simulink model "SimulinkModel"  (R2026a)
settings: Solver=ode23s  StopTime=5
values from neighbouring files (symbols this model uses):
  Kd = 2    [BaseSkript.m]
  Ki = 1.5    [BaseSkript.m]
  Kp = 40    [BaseSkript.m]
  Nd = 100    [BaseSkript.m]    (also in Master_Combination_Run.m; Master_Combination_Run_Prisme.m)
  s = 10*tau^3 - 15*tau^4 + 6*tau^5    [Math_Model.m]    (also in calculate_delta_torque.m = u^3 * (10 - 15*u + 6*u^2))
  X = P(1)*cos(phi_ang) + P(2)*sin(phi_ang)    [Math_Model.m]    (also in calculate_delta_torque.m = P(1)*cos(phi) + P(2)*sin(phi))
  Y = -P(1)*sin(phi_ang) + P(2)*cos(phi_ang)    [Math_Model.m]    (also in calculate_delta_torque.m = -P(1)*sin(phi) + P(2)*cos(phi))
  Z = P(3)    [Math_Model.m]    (also in calculate_delta_torque.m)
undefined symbols (not defined in the file or in its folder): params
libraries: sm_lib x17, nesl_utility x13, slpidlib x3
settings Model: Creator=louis  LastModifiedBy=louis

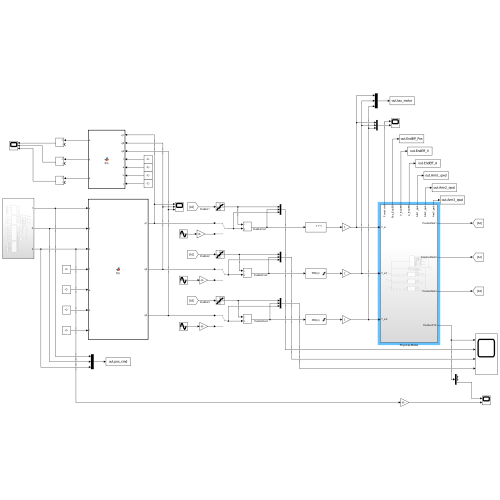
[thumbnail: Simulink's stored preview of the top-level diagram]
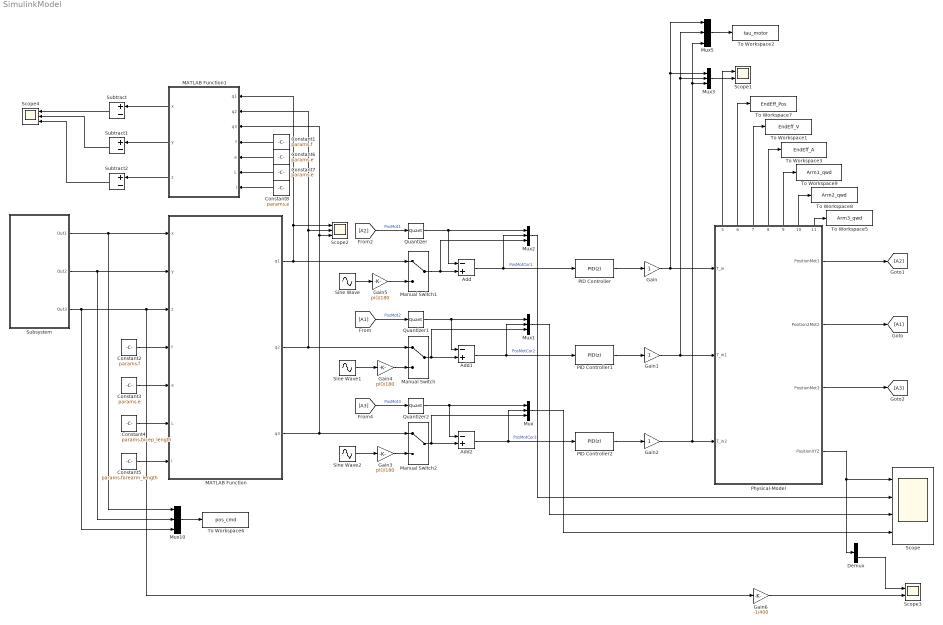
== system SimulinkModel ==
  Add : Sum  Inputs=-+
  Add1 : Sum  Inputs=-+
  Add2 : Sum  Inputs=-+
  Constant1 : Constant  Value=params.f
  Constant2 : Constant  Value=params.f
  Constant{3,6..8} (4 alike) : Constant  Value=params.e
  Constant4 : Constant  Value=params.bicep_length
  Constant5 : Constant  Value=params.forearm_length
  Demux : Demux  Outputs=3
  Gain : Gain
  Gain1 : Gain
  Gain2 : Gain
  Gain3 : Gain  Gain=pi()/180
  Gain4 : Gain  Gain=pi()/180
  Gain5 : Gain  Gain=pi()/180
  Gain6 : Gain  Gain=-1/400
  MATLAB Function : MATLAB Function  TreatAsAtomicUnit=on
  MATLAB Function1 : MATLAB Function  TreatAsAtomicUnit=on
  Manual Switch : ManualSwitch
  Manual Switch1 : ManualSwitch
  Manual Switch2 : ManualSwitch
  Mux{,1..3,5,10} (6 alike) : Mux  Inputs=3
  PID Controller : slpidlib/PID Controller  Controller=PID  Form=Parallel  TimeDomain=Discrete-time  UseExternalTs=off  SampleTime=0.001  IntegratorMethod=Forward Euler  FilterMethod=Forward Euler  ControllerParametersSource=internal  P=Kp  I=Ki  UseKiTs=off  D=Kd  UseExternalDerivativeSource=off  N=Nd  UseFilter=on  TunerSelectOption=Transfer Function Based (PID Tuner App)  InitialConditionSource=internal  InitialConditionForIntegrator=0  InitialConditionForFilter=0  DifferentiatorICPrevScaledInput=0  ExternalReset=none  TrackingMode=off  Kt=1  LimitOutput=on  SatLimitsSource=internal  UpperSaturationLimit=params.saturation_tau  LowerSaturationLimit=-params.saturation_tau  LinearizeAsGain=on  AntiWindupMode=none  Kb=1  LimitIntegrator=off  UpperIntegratorSaturationLimit=inf  LowerIntegratorSaturationLimit=-inf  POutMin=[]  POutMax=[]  IOutMin=[]  IOutMax=[]  DOutMin=[]  DOutMax=[]  NOutMin=[]  NOutMax=[]  SumOutMin=[]  SumOutMax=[]  SaturationOutMin=[]  SaturationOutMax=[]  PParamMin=[]  PParamMax=[]  IParamMin=[]  IParamMax=[]  DParamMin=[]  DParamMax=[]  NParamMin=[]  NParamMax=[]  KbParamMin=[]  KbParamMax=[]  KtParamMin=[]  KtParamMax=[]  KbOutMin=[]  KbOutMax=[]  KtOutMin=[]  KtOutMax=[]  IntegratorOutMin=[]  IntegratorOutMax=[]  FilterOutMin=[]  FilterOutMax=[]  SumI1OutMin=[]  SumI1OutMax=[]  SumI2OutMin=[]  SumI2OutMax=[]  SumI3OutMin=[]  SumI3OutMax=[]  SumI4OutMin=[]  SumI4OutMax=[]  SumDOutMin=[]  SumDOutMax=[]  DifferentiatorOutMin=[]  DifferentiatorOutMax=[]  FilterDiffOutCoefMin=[]  FilterDiffOutCoefMax=[]  ReciprocalOutMin=[]  ReciprocalOutMax=[]  SumDenOutMin=[]  SumDenOutMax=[]  SumNumOutMin=[]  SumNumOutMax=[]  DivideOutMin=[]  DivideOutMax=[]  UdiffTsProdOutMin=[]  UdiffTsProdOutMax=[]  NTsProdOutMin=[]  NTsProdOutMax=[]  UintegralTsProdOutMin=[]  UintegralTsProdOutMax=[]  UngainTsProdOutMin=[]  UngainTsProdOutMax=[]  ClampingZeroOutDataTypeStr=Inherit: Inherit via back propagation  ClampingZeroOutMin=[]  ClampingZeroOutMax=[]  FilterDenConstantOutDataTypeStr=Inherit: Inherit via back propagation  FilterDenConstantOutMin=[]  FilterDenConstantOutMax=[]  PCopyOutDataTypeStr=Inherit: Inherit via back propagation  PCopyOutMin=[]  PCopyOutMax=[]  NCopyOutDataTypeStr=Inherit: Inherit via back propagation  NCopyOutMin=[]  NCopyOutMax=[]  IntegratorContinuousStateAttributes=''  IntegratorStateMustResolveToSignalObject=off  IntegratorRTWStateStorageClass=Auto  FilterContinuousStateAttributes=''  FilterStateMustResolveToSignalObject=off  FilterRTWStateStorageClass=Auto  ParallelPVariant=InternalParameters  IdealPVariant=Disabled  IVariant=InternalParameters  DVariant=InternalParameters  IntegratorVariant=Discrete  SatVariant=Enabled  AWVariant=Passthrough  PCopyVariant=Disabled  TRVariant=Disabled  FdbkBlocksVariant=Forward  IdealPFdbkVariant=Disabled  SatFdbkVariant=Disabled  DerivativeFilterVariant=ForwardEulerFilter  NVariant=InternalParameters  NCopyVariant=Disabled  FilterICVariant=InternalICsFilter  IntegratorICVariant=InternalICs  ExternalResetVariant=Disabled  TRSumVariant=Passthrough  SumFdbkVariant=Disabled  SumVariant=Sum_PID  TsampFilterVariant=InternalTs  TsampNgainVariant=Passthrough  TsampIntegralVariant=Disabled_SignalSpec  ExternalSaturationOutDataTypeStr=Inherit: Same as second input  DerivativeSourceVariant=ErrorSignal  PreIntVariant=InternalPreInt
  PID Controller1 : slpidlib/PID Controller  Controller=PID  Form=Parallel  TimeDomain=Discrete-time  UseExternalTs=off  SampleTime=0.001  IntegratorMethod=Forward Euler  FilterMethod=Forward Euler  ControllerParametersSource=internal  P=Kp  I=Ki  UseKiTs=off  D=Kd  UseExternalDerivativeSource=off  N=Nd  UseFilter=on  TunerSelectOption=Transfer Function Based (PID Tuner App)  InitialConditionSource=internal  InitialConditionForIntegrator=0  InitialConditionForFilter=0  DifferentiatorICPrevScaledInput=0  ExternalReset=none  TrackingMode=off  Kt=1  LimitOutput=on  SatLimitsSource=internal  UpperSaturationLimit=params.saturation_tau  LowerSaturationLimit=-params.saturation_tau  LinearizeAsGain=on  AntiWindupMode=none  Kb=1  LimitIntegrator=off  UpperIntegratorSaturationLimit=inf  LowerIntegratorSaturationLimit=-inf  POutMin=[]  POutMax=[]  IOutMin=[]  IOutMax=[]  DOutMin=[]  DOutMax=[]  NOutMin=[]  NOutMax=[]  SumOutMin=[]  SumOutMax=[]  SaturationOutMin=[]  SaturationOutMax=[]  PParamMin=[]  PParamMax=[]  IParamMin=[]  IParamMax=[]  DParamMin=[]  DParamMax=[]  NParamMin=[]  NParamMax=[]  KbParamMin=[]  KbParamMax=[]  KtParamMin=[]  KtParamMax=[]  KbOutMin=[]  KbOutMax=[]  KtOutMin=[]  KtOutMax=[]  IntegratorOutMin=[]  IntegratorOutMax=[]  FilterOutMin=[]  FilterOutMax=[]  SumI1OutMin=[]  SumI1OutMax=[]  SumI2OutMin=[]  SumI2OutMax=[]  SumI3OutMin=[]  SumI3OutMax=[]  SumI4OutMin=[]  SumI4OutMax=[]  SumDOutMin=[]  SumDOutMax=[]  DifferentiatorOutMin=[]  DifferentiatorOutMax=[]  FilterDiffOutCoefMin=[]  FilterDiffOutCoefMax=[]  ReciprocalOutMin=[]  ReciprocalOutMax=[]  SumDenOutMin=[]  SumDenOutMax=[]  SumNumOutMin=[]  SumNumOutMax=[]  DivideOutMin=[]  DivideOutMax=[]  UdiffTsProdOutMin=[]  UdiffTsProdOutMax=[]  NTsProdOutMin=[]  NTsProdOutMax=[]  UintegralTsProdOutMin=[]  UintegralTsProdOutMax=[]  UngainTsProdOutMin=[]  UngainTsProdOutMax=[]  ClampingZeroOutDataTypeStr=Inherit: Inherit via back propagation  ClampingZeroOutMin=[]  ClampingZeroOutMax=[]  FilterDenConstantOutDataTypeStr=Inherit: Inherit via back propagation  FilterDenConstantOutMin=[]  FilterDenConstantOutMax=[]  PCopyOutDataTypeStr=Inherit: Inherit via back propagation  PCopyOutMin=[]  PCopyOutMax=[]  NCopyOutDataTypeStr=Inherit: Inherit via back propagation  NCopyOutMin=[]  NCopyOutMax=[]  IntegratorContinuousStateAttributes=''  IntegratorStateMustResolveToSignalObject=off  IntegratorRTWStateStorageClass=Auto  FilterContinuousStateAttributes=''  FilterStateMustResolveToSignalObject=off  FilterRTWStateStorageClass=Auto  ParallelPVariant=InternalParameters  IdealPVariant=Disabled  IVariant=InternalParameters  DVariant=InternalParameters  IntegratorVariant=Discrete  SatVariant=Enabled  AWVariant=Passthrough  PCopyVariant=Disabled  TRVariant=Disabled  FdbkBlocksVariant=Forward  IdealPFdbkVariant=Disabled  SatFdbkVariant=Disabled  DerivativeFilterVariant=ForwardEulerFilter  NVariant=InternalParameters  NCopyVariant=Disabled  FilterICVariant=InternalICsFilter  IntegratorICVariant=InternalICs  ExternalResetVariant=Disabled  TRSumVariant=Passthrough  SumFdbkVariant=Disabled  SumVariant=Sum_PID  TsampFilterVariant=InternalTs  TsampNgainVariant=Passthrough  TsampIntegralVariant=Disabled_SignalSpec  ExternalSaturationOutDataTypeStr=Inherit: Same as second input  DerivativeSourceVariant=ErrorSignal  PreIntVariant=InternalPreInt
  PID Controller2 : slpidlib/PID Controller  Controller=PID  Form=Parallel  TimeDomain=Discrete-time  UseExternalTs=off  SampleTime=0.001  IntegratorMethod=Forward Euler  FilterMethod=Forward Euler  ControllerParametersSource=internal  P=Kp  I=Ki  UseKiTs=off  D=Kd  UseExternalDerivativeSource=off  N=Nd  UseFilter=on  TunerSelectOption=Transfer Function Based (PID Tuner App)  InitialConditionSource=internal  InitialConditionForIntegrator=0.2  InitialConditionForFilter=0.2  DifferentiatorICPrevScaledInput=0  ExternalReset=none  TrackingMode=off  Kt=1  LimitOutput=on  SatLimitsSource=internal  UpperSaturationLimit=params.saturation_tau  LowerSaturationLimit=-params.saturation_tau  LinearizeAsGain=on  AntiWindupMode=none  Kb=1  LimitIntegrator=off  UpperIntegratorSaturationLimit=inf  LowerIntegratorSaturationLimit=-inf  POutMin=[]  POutMax=[]  IOutMin=[]  IOutMax=[]  DOutMin=[]  DOutMax=[]  NOutMin=[]  NOutMax=[]  SumOutMin=[]  SumOutMax=[]  SaturationOutMin=[]  SaturationOutMax=[]  PParamMin=[]  PParamMax=[]  IParamMin=[]  IParamMax=[]  DParamMin=[]  DParamMax=[]  NParamMin=[]  NParamMax=[]  KbParamMin=[]  KbParamMax=[]  KtParamMin=[]  KtParamMax=[]  KbOutMin=[]  KbOutMax=[]  KtOutMin=[]  KtOutMax=[]  IntegratorOutMin=[]  IntegratorOutMax=[]  FilterOutMin=[]  FilterOutMax=[]  SumI1OutMin=[]  SumI1OutMax=[]  SumI2OutMin=[]  SumI2OutMax=[]  SumI3OutMin=[]  SumI3OutMax=[]  SumI4OutMin=[]  SumI4OutMax=[]  SumDOutMin=[]  SumDOutMax=[]  DifferentiatorOutMin=[]  DifferentiatorOutMax=[]  FilterDiffOutCoefMin=[]  FilterDiffOutCoefMax=[]  ReciprocalOutMin=[]  ReciprocalOutMax=[]  SumDenOutMin=[]  SumDenOutMax=[]  SumNumOutMin=[]  SumNumOutMax=[]  DivideOutMin=[]  DivideOutMax=[]  UdiffTsProdOutMin=[]  UdiffTsProdOutMax=[]  NTsProdOutMin=[]  NTsProdOutMax=[]  UintegralTsProdOutMin=[]  UintegralTsProdOutMax=[]  UngainTsProdOutMin=[]  UngainTsProdOutMax=[]  ClampingZeroOutDataTypeStr=Inherit: Inherit via back propagation  ClampingZeroOutMin=[]  ClampingZeroOutMax=[]  FilterDenConstantOutDataTypeStr=Inherit: Inherit via back propagation  FilterDenConstantOutMin=[]  FilterDenConstantOutMax=[]  PCopyOutDataTypeStr=Inherit: Inherit via back propagation  PCopyOutMin=[]  PCopyOutMax=[]  NCopyOutDataTypeStr=Inherit: Inherit via back propagation  NCopyOutMin=[]  NCopyOutMax=[]  IntegratorContinuousStateAttributes=''  IntegratorStateMustResolveToSignalObject=off  IntegratorRTWStateStorageClass=Auto  FilterContinuousStateAttributes=''  FilterStateMustResolveToSignalObject=off  FilterRTWStateStorageClass=Auto  ParallelPVariant=InternalParameters  IdealPVariant=Disabled  IVariant=InternalParameters  DVariant=InternalParameters  IntegratorVariant=Discrete  SatVariant=Enabled  AWVariant=Passthrough  PCopyVariant=Disabled  TRVariant=Disabled  FdbkBlocksVariant=Forward  IdealPFdbkVariant=Disabled  SatFdbkVariant=Disabled  DerivativeFilterVariant=ForwardEulerFilter  NVariant=InternalParameters  NCopyVariant=Disabled  FilterICVariant=InternalICsFilter  IntegratorICVariant=InternalICs  ExternalResetVariant=Disabled  TRSumVariant=Passthrough  SumFdbkVariant=Disabled  SumVariant=Sum_PID  TsampFilterVariant=InternalTs  TsampNgainVariant=Passthrough  TsampIntegralVariant=Disabled_SignalSpec  ExternalSaturationOutDataTypeStr=Inherit: Same as second input  DerivativeSourceVariant=ErrorSignal  PreIntVariant=InternalPreInt
  Physical-Model : Subsystem
      settings: PortSchema="{\"entries\":[{\"content\":{\"sides\":[{\"content\":{\"connectorIds\":[\"In1\",\"In2\",\"In3\"]},\"type\":\"ConnectorPlacement.EquallySpacedRectSide\",\"uuid\":\"472b42dc-ef62-4194-8627-c0d485c40d23\"},{\"content\":{\"connectorIds\":[\"Out1\",\"Out2\",\"Out3\",\"Out4\"],\"side\":\"RIGHT\"},\"type\":\"ConnectorPlacement.EquallySpacedRectSide\",\"uuid\":\"1afa02f3-9060-449b-bf9c-19485df79b48\"},{\"content\":{\"connectorIds\":[\"Out5\",\"Out6\",\"Out7\",\"Out8\",\"Out9\",\"Out10\",\"Out11\"],\"side\":\"TOP\"},\"type\":\"ConnectorPlacement.EquallySpacedRectSide\",\"uuid\":\"4b06c459-0470-40e7-9b6b-03b6062bc28f\"}]},\"type\":\"ConnectorPlacement.EquallySpacedConnector\",\"uuid\":\"0d09a3c9-0e0a-4c94-88b6-5aaedb495534\"}],\"packageUris\":[\"http://schema.mathworks.com/mf0/Connector/R2020b\"],\"version\":\"1.0\"}"
  Quantizer : Quantizer  QuantizationInterval=(2*pi())/params.pulses_per_rev
  Quantizer1 : Quantizer  QuantizationInterval=(2*pi())/params.pulses_per_rev
  Quantizer2 : Quantizer  QuantizationInterval=(2*pi())/params.pulses_per_rev
  Scope : Scope  NumInputPorts=4
      settings: ActiveDisplayYMinimum=-0.346817893581086  ActiveDisplayYMaximum=0.17909621572480147
  Scope1 : Scope  NumInputPorts=2
      settings: ActiveDisplayYMinimum=-518.62097461648136  ActiveDisplayYMaximum=668.9682157183538
  Scope2 : Scope  NumInputPorts=3
      settings: ActiveDisplayYMinimum=0.80317985150487559  ActiveDisplayYMaximum=1.6546987147027221  DataLoggingVariableName=ScopeData2
  Scope3 : Scope  NumInputPorts=2
      settings: ActiveDisplayYMinimum=-0.36067756279258084  ActiveDisplayYMaximum=-0.28326753588358305  DataLoggingVariableName=ScopeData3
  Scope4 : Scope  NumInputPorts=3
      settings: ActiveDisplayYMinimum=-48.031147138395717  ActiveDisplayYMaximum=34.968785901954071  DataLoggingVariableName=ScopeData4
  Sine Wave : Sin  Amplitude=30  Bias=70  Frequency=2*pi()*2  Phase=(3/3) *( 2*pi())  SampleTime=0
  Sine Wave1 : Sin  Amplitude=30  Bias=70  Frequency=2*pi()*2  Phase=(1/3) *(2* pi())  SampleTime=0
  Sine Wave2 : Sin  Amplitude=30  Bias=70  Frequency=2*pi()*2  Phase=(2/3) *( 2*pi())  SampleTime=0
  Subsystem : Subsystem
  Subtract : Sum  Inputs=+-
  Subtract1 : Sum  Inputs=+-
  Subtract2 : Sum  Inputs=+-
  To Workspace1 : ToWorkspace  VariableName=EndEff_V  SaveFormat=Timeseries  SampleTime=-1
  To Workspace2 : ToWorkspace  VariableName=tau_motor  SaveFormat=Timeseries  SampleTime=-1
  To Workspace3 : ToWorkspace  VariableName=EndEff_A  SaveFormat=Timeseries  SampleTime=-1
  To Workspace5 : ToWorkspace  VariableName=Arm3_qwd  SaveFormat=Timeseries  SampleTime=-1
  To Workspace6 : ToWorkspace  VariableName=pos_cmd  SaveFormat=Timeseries  SampleTime=-1
  To Workspace7 : ToWorkspace  VariableName=EndEff_Pos  SaveFormat=Timeseries  SampleTime=-1
  To Workspace8 : ToWorkspace  VariableName=Arm2_qwd  SaveFormat=Timeseries  SampleTime=-1
  To Workspace9 : ToWorkspace  VariableName=Arm1_qwd  SaveFormat=Timeseries  SampleTime=-1
  wires:
  Add/1 -> PID Controller/1, Mux2/2  "PosMotCor1"
  Add2/1 -> PID Controller2/1, Mux/2  "PosMotCor3"
  Add1/1 -> PID Controller1/1, Mux1/2  "PosMotCor2"
  [A1] -> Quantizer1/1  "PosMot2"
  [A2] -> Quantizer/1  "PosMot1"
  [A3] -> Quantizer2/1  "PosMot3"
  Mux2/1 -> Scope/2
  Mux1/1 -> Scope/3
  Mux/1 -> Scope/4
  Constant3/1 -> MATLAB Function/5(e)
  Constant2/1 -> MATLAB Function/4(f)
  Constant4/1 -> MATLAB Function/6(L)
  Constant5/1 -> MATLAB Function/7(l)
  Gain/1 -> Physical-Model/1(T_in), Mux3/1, Mux5/1
  Gain1/1 -> Physical-Model/2(T_in1), Mux3/2, Mux5/2
  Gain2/1 -> Physical-Model/3(T_in2), Mux5/3, Mux3/3
  MATLAB Function/1(q1) -> MATLAB Function1/1(q1), Scope2/1, Manual Switch1/1
  MATLAB Function/3(q3) -> Manual Switch2/1, MATLAB Function1/3(q3), Scope2/3
  MATLAB Function/2(q2) -> Manual Switch/1, MATLAB Function1/2(q2), Scope2/2
  PID Controller/1 -> Gain/1
  PID Controller1/1 -> Gain1/1
  Sine Wave/1 -> Gain5/1
  Sine Wave1/1 -> Gain4/1
  Sine Wave2/1 -> Gain3/1
  PID Controller2/1 -> Gain2/1
  Gain4/1 -> Manual Switch/2
  Manual Switch1/1 -> Mux2/3, Add/2
  Gain5/1 -> Manual Switch1/2
  Manual Switch2/1 -> Mux/3, Add2/2
  Gain3/1 -> Manual Switch2/2
  Manual Switch/1 -> Mux1/3, Add1/2
  Subsystem/1(Out1) -> MATLAB Function/1(x), Mux10/1
  Subsystem/2(Out2) -> MATLAB Function/2(y), Mux10/2
  Subsystem/3(Out3) -> Mux10/3, MATLAB Function/3(z), Gain6/1
  Quantizer/1 -> Add/1, Mux2/1
  Quantizer1/1 -> Mux1/1, Add1/1
  Quantizer2/1 -> Mux/1, Add2/1
  Gain6/1 -> Scope3/2
  Demux/3 -> Scope3/1
  Constant1/1 -> MATLAB Function1/4(f)
  Constant6/1 -> MATLAB Function1/5(e)
  Constant7/1 -> MATLAB Function1/6(L)
  Constant8/1 -> MATLAB Function1/7(l)
  MATLAB Function1/1(x) -> Subtract/1
  MATLAB Function1/2(y) -> Subtract1/1
  MATLAB Function1/3(z) -> Subtract2/1
  Subtract/1 -> Scope4/1
  Subtract1/1 -> Scope4/2
  Subtract2/1 -> Scope4/3
  Mux3/1 -> Scope1/2
  Physical-Model/1(PositionMot1) -> [A2]
  Physical-Model/2(Position2Mot2) -> [A1]
  Physical-Model/3(PositionMot3) -> [A3]
  Physical-Model/4(PositionXYZ) -> Scope/1, Demux/1
  Physical-Model/5(ForceJoint) -> Scope1/1
  Mux10/1 -> To Workspace6/1
  Physical-Model/8(A_EndEff) -> To Workspace3/1
  Physical-Model/11(Arm3_qwb) -> To Workspace5/1
  Mux5/1 -> To Workspace2/1
  Physical-Model/7(V_EndEff) -> To Workspace1/1
  Physical-Model/6(Pos_EndEff) -> To Workspace7/1
  Physical-Model/10(Arm2_qwb) -> To Workspace8/1
  Physical-Model/9(Arm1_qwb) -> To Workspace9/1

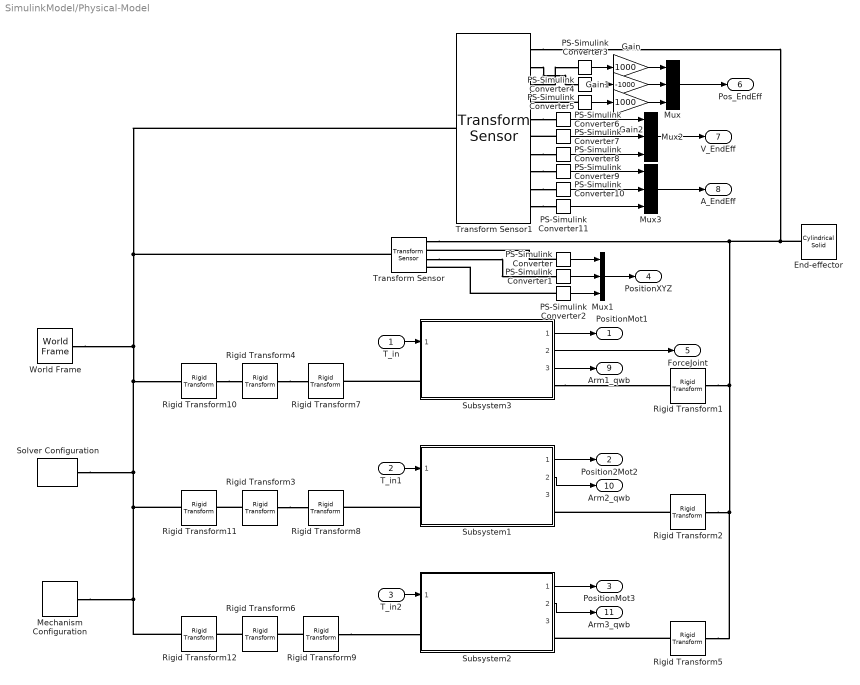
== system SimulinkModel/Physical-Model ==
  T_in : Inport
  T_in1 : Inport  Port=2
  T_in2 : Inport  Port=3
  End-effector : sm_lib/Body Elements/Cylindrical Solid  CylinderRadius=params.plate_radius  CylinderRadiusUnits=mm  CylinderLength=params.plate_thickness  CylinderLengthUnits=mm  ExportEntireGeometry=off  InertiaType=CalculateFromGeometry  BasedOnType=Density  Density=params.rho_aluminum  DensityUnits=kg/m^3  Mass=1  MassUnits=kg  CenterOfMass=[0 0 0]  CenterOfMassUnits=m  MomentsOfInertia=[1 1 1]  MomentsOfInertiaUnits=kg*m^2  ProductsOfInertia=[0 0 0]  ProductsOfInertiaUnits=kg*m^2  GraphicType=FromGeometry  MarkerShape=Sphere  MarkerSize=10  GraphicVisPropType=SimpleVisualProperties  GraphicDiffuseColor=[0 0.3333 1]  GraphicOpacity=1  GraphicSpecularColor=[0.5 0.5 0.5 1.0]  GraphicAmbientColor=[0.15 0.15 0.15 1.0]  GraphicEmissiveColor=[0.0 0.0 0.0 1.0]  GraphicShininess=75  DoExposeReferenceFrame=off  SerializedFrames=<Frames><Frame><Id>Frame1</Id><Value><Name>F1</Name><Origin><Source>GeometricFeature</Source><FeatureName>top surface</FeatureName></Origin><PrimaryAxis><DefinedDirection>+Z</DefinedDirection><Source>ReferenceFrame</Source><SourceDirection>+Z</SourceDirection><FeatureName></FeatureName></PrimaryAxis><SecondaryAxis><DefinedDirection>+X</DefinedDirection><Source>ReferenceFrame</Source><SourceDirection>+X</SourceDirection><FeatureName></FeatureName></SecondaryAxis></Value></Frame></Frames>
  Gain : Gain  Gain=1000
  Gain1 : Gain  Gain=-1000
  Gain2 : Gain  Gain=1000
  Mechanism Configuration : sm_lib/Utilities/Mechanism Configuration  UniformGravity=Constant  GravityVector=[0 0 -9.81]  GravityVectorUnits=m/s^2  LinearizationDelta=0.001  JointModeTransitionNonlinearIterations=2
  Mux{,1..3} (4 alike) : Mux  Inputs=3
  PS-Simulink Converter{,1..11} (12 alike) : nesl_utility/PS-Simulink Converter  PhysicalDomain=network_engine_domain  SubClassName=ps_output  LeftPortType=input  RightPortType=output  PseudoPeriodic=off  Frequencies=[]  VectorFormat=inherit  Unit=inherit  AffineConversion=off
  Rigid Transform1 : sm_lib/Frames and Transforms/Rigid Transform  RotationMethod=StandardAxis  FollAlignAxisA=+X  BaseAlignAxisA=+Y  FollAlignAxisB=+Y  BaseAlignAxisB=+Z  RotationStandardAxis=+Z  RotationAngle=0  RotationAngleUnits=deg  RotationArbitraryAxis=[0 0 1]  RotationSequenceAxes=FollowerAxes  RotationSequence=XYX  RotationSequenceAngles=[0 0 0]  RotationSequenceAnglesUnits=deg  RotationMatrix=[1 0 0;0 1 0;0 0 1]  Quaternion=[1 0 0 0]  TranslationMethod=Cartesian  TranslationCartesianOffset=[params.plate_radius 0 0]  TranslationCartesianOffsetUnits=mm  TranslationStandardAxis=+Z  TranslationStandardOffset=0  TranslationStandardOffsetUnits=m  TranslationROffset=0  TranslationROffsetUnits=m  TranslationThetaOffset=0  TranslationThetaOffsetUnits=deg  TranslationZOffset=0  TranslationZOffsetUnits=m
  Rigid Transform10 : sm_lib/Frames and Transforms/Rigid Transform  RotationMethod=StandardAxis  FollAlignAxisA=+X  BaseAlignAxisA=+Y  FollAlignAxisB=+Y  BaseAlignAxisB=+Z  RotationStandardAxis=+X  RotationAngle=180  RotationAngleUnits=deg  RotationArbitraryAxis=[0 0 1]  RotationSequenceAxes=FollowerAxes  RotationSequence=XYX  RotationSequenceAngles=[0 0 0]  RotationSequenceAnglesUnits=deg  RotationMatrix=[1 0 0;0 1 0;0 0 1]  Quaternion=[1 0 0 0]  TranslationMethod=None  TranslationCartesianOffset=[params.f 0 0]  TranslationCartesianOffsetUnits=mm  TranslationStandardAxis=+Z  TranslationStandardOffset=0  TranslationStandardOffsetUnits=m  TranslationROffset=0  TranslationROffsetUnits=m  TranslationThetaOffset=0  TranslationThetaOffsetUnits=deg  TranslationZOffset=0  TranslationZOffsetUnits=m
  Rigid Transform11 : sm_lib/Frames and Transforms/Rigid Transform  RotationMethod=StandardAxis  FollAlignAxisA=+X  BaseAlignAxisA=+Y  FollAlignAxisB=+Y  BaseAlignAxisB=+Z  RotationStandardAxis=+X  RotationAngle=180  RotationAngleUnits=deg  RotationArbitraryAxis=[0 0 1]  RotationSequenceAxes=FollowerAxes  RotationSequence=XYX  RotationSequenceAngles=[0 0 0]  RotationSequenceAnglesUnits=deg  RotationMatrix=[1 0 0;0 1 0;0 0 1]  Quaternion=[1 0 0 0]  TranslationMethod=None  TranslationCartesianOffset=[params.f 0 0]  TranslationCartesianOffsetUnits=mm  TranslationStandardAxis=+Z  TranslationStandardOffset=0  TranslationStandardOffsetUnits=m  TranslationROffset=0  TranslationROffsetUnits=m  TranslationThetaOffset=0  TranslationThetaOffsetUnits=deg  TranslationZOffset=0  TranslationZOffsetUnits=m
  Rigid Transform12 : sm_lib/Frames and Transforms/Rigid Transform  RotationMethod=StandardAxis  FollAlignAxisA=+X  BaseAlignAxisA=+Y  FollAlignAxisB=+Y  BaseAlignAxisB=+Z  RotationStandardAxis=+X  RotationAngle=180  RotationAngleUnits=deg  RotationArbitraryAxis=[0 0 1]  RotationSequenceAxes=FollowerAxes  RotationSequence=XYX  RotationSequenceAngles=[0 0 0]  RotationSequenceAnglesUnits=deg  RotationMatrix=[1 0 0;0 1 0;0 0 1]  Quaternion=[1 0 0 0]  TranslationMethod=None  TranslationCartesianOffset=[params.f 0 0]  TranslationCartesianOffsetUnits=mm  TranslationStandardAxis=+Z  TranslationStandardOffset=0  TranslationStandardOffsetUnits=m  TranslationROffset=0  TranslationROffsetUnits=m  TranslationThetaOffset=0  TranslationThetaOffsetUnits=deg  TranslationZOffset=0  TranslationZOffsetUnits=m
  Rigid Transform2 : sm_lib/Frames and Transforms/Rigid Transform  RotationMethod=StandardAxis  FollAlignAxisA=+X  BaseAlignAxisA=+Y  FollAlignAxisB=+Y  BaseAlignAxisB=+Z  RotationStandardAxis=+Z  RotationAngle=-120  RotationAngleUnits=deg  RotationArbitraryAxis=[0 0 1]  RotationSequenceAxes=FollowerAxes  RotationSequence=XYX  RotationSequenceAngles=[0 0 0]  RotationSequenceAnglesUnits=deg  RotationMatrix=[1 0 0;0 1 0;0 0 1]  Quaternion=[1 0 0 0]  TranslationMethod=Cartesian  TranslationCartesianOffset=[params.plate_radius 0 0]  TranslationCartesianOffsetUnits=mm  TranslationStandardAxis=+Z  TranslationStandardOffset=0  TranslationStandardOffsetUnits=m  TranslationROffset=0  TranslationROffsetUnits=m  TranslationThetaOffset=0  TranslationThetaOffsetUnits=deg  TranslationZOffset=0  TranslationZOffsetUnits=m
  Rigid Transform3 : sm_lib/Frames and Transforms/Rigid Transform  RotationMethod=StandardAxis  FollAlignAxisA=+X  BaseAlignAxisA=+Y  FollAlignAxisB=+Y  BaseAlignAxisB=+Z  RotationStandardAxis=+Z  RotationAngle=-120  RotationAngleUnits=deg  RotationArbitraryAxis=[0 0 1]  RotationSequenceAxes=FollowerAxes  RotationSequence=XYX  RotationSequenceAngles=[0 0 0]  RotationSequenceAnglesUnits=deg  RotationMatrix=[1 0 0;0 1 0;0 0 1]  Quaternion=[1 0 0 0]  TranslationMethod=None  TranslationCartesianOffset=[params.f 0 0]  TranslationCartesianOffsetUnits=mm  TranslationStandardAxis=+Z  TranslationStandardOffset=0  TranslationStandardOffsetUnits=m  TranslationROffset=0  TranslationROffsetUnits=m  TranslationThetaOffset=0  TranslationThetaOffsetUnits=deg  TranslationZOffset=0  TranslationZOffsetUnits=m
  Rigid Transform4 : sm_lib/Frames and Transforms/Rigid Transform  RotationMethod=StandardAxis  FollAlignAxisA=+X  BaseAlignAxisA=+Y  FollAlignAxisB=+Y  BaseAlignAxisB=+Z  RotationStandardAxis=+Z  RotationAngle=0  RotationAngleUnits=deg  RotationArbitraryAxis=[0 0 1]  RotationSequenceAxes=FollowerAxes  RotationSequence=XYX  RotationSequenceAngles=[0 0 0]  RotationSequenceAnglesUnits=deg  RotationMatrix=[1 0 0;0 1 0;0 0 1]  Quaternion=[1 0 0 0]  TranslationMethod=None  TranslationCartesianOffset=[params.f 0 0]  TranslationCartesianOffsetUnits=mm  TranslationStandardAxis=+Z  TranslationStandardOffset=0  TranslationStandardOffsetUnits=m  TranslationROffset=0  TranslationROffsetUnits=m  TranslationThetaOffset=0  TranslationThetaOffsetUnits=deg  TranslationZOffset=0  TranslationZOffsetUnits=m
  Rigid Transform5 : sm_lib/Frames and Transforms/Rigid Transform  RotationMethod=StandardAxis  FollAlignAxisA=+X  BaseAlignAxisA=+Y  FollAlignAxisB=+Y  BaseAlignAxisB=+Z  RotationStandardAxis=+Z  RotationAngle=120  RotationAngleUnits=deg  RotationArbitraryAxis=[0 0 1]  RotationSequenceAxes=FollowerAxes  RotationSequence=XYX  RotationSequenceAngles=[0 0 0]  RotationSequenceAnglesUnits=deg  RotationMatrix=[1 0 0;0 1 0;0 0 1]  Quaternion=[1 0 0 0]  TranslationMethod=Cartesian  TranslationCartesianOffset=[params.plate_radius 0 0]  TranslationCartesianOffsetUnits=mm  TranslationStandardAxis=+Z  TranslationStandardOffset=0  TranslationStandardOffsetUnits=m  TranslationROffset=0  TranslationROffsetUnits=m  TranslationThetaOffset=0  TranslationThetaOffsetUnits=deg  TranslationZOffset=0  TranslationZOffsetUnits=m
  Rigid Transform6 : sm_lib/Frames and Transforms/Rigid Transform  RotationMethod=StandardAxis  FollAlignAxisA=+X  BaseAlignAxisA=+Y  FollAlignAxisB=+Y  BaseAlignAxisB=+Z  RotationStandardAxis=+Z  RotationAngle=120  RotationAngleUnits=deg  RotationArbitraryAxis=[0 0 1]  RotationSequenceAxes=FollowerAxes  RotationSequence=XYX  RotationSequenceAngles=[0 0 0]  RotationSequenceAnglesUnits=deg  RotationMatrix=[1 0 0;0 1 0;0 0 1]  Quaternion=[1 0 0 0]  TranslationMethod=None  TranslationCartesianOffset=[params.f 0 0]  TranslationCartesianOffsetUnits=mm  TranslationStandardAxis=+Z  TranslationStandardOffset=0  TranslationStandardOffsetUnits=m  TranslationROffset=0  TranslationROffsetUnits=m  TranslationThetaOffset=0  TranslationThetaOffsetUnits=deg  TranslationZOffset=0  TranslationZOffsetUnits=m
  Rigid Transform7 : sm_lib/Frames and Transforms/Rigid Transform  RotationMethod=None  FollAlignAxisA=+X  BaseAlignAxisA=+Y  FollAlignAxisB=+Y  BaseAlignAxisB=+Z  RotationStandardAxis=+Z  RotationAngle=0  RotationAngleUnits=deg  RotationArbitraryAxis=[0 0 1]  RotationSequenceAxes=FollowerAxes  RotationSequence=XYX  RotationSequenceAngles=[0 0 0]  RotationSequenceAnglesUnits=deg  RotationMatrix=[1 0 0;0 1 0;0 0 1]  Quaternion=[1 0 0 0]  TranslationMethod=Cartesian  TranslationCartesianOffset=[params.f 0 0]  TranslationCartesianOffsetUnits=mm  TranslationStandardAxis=+Z  TranslationStandardOffset=0  TranslationStandardOffsetUnits=m  TranslationROffset=0  TranslationROffsetUnits=m  TranslationThetaOffset=0  TranslationThetaOffsetUnits=deg  TranslationZOffset=0  TranslationZOffsetUnits=m
  Rigid Transform8 : sm_lib/Frames and Transforms/Rigid Transform  RotationMethod=None  FollAlignAxisA=+X  BaseAlignAxisA=+Y  FollAlignAxisB=+Y  BaseAlignAxisB=+Z  RotationStandardAxis=+Z  RotationAngle=0  RotationAngleUnits=deg  RotationArbitraryAxis=[0 0 1]  RotationSequenceAxes=FollowerAxes  RotationSequence=XYX  RotationSequenceAngles=[0 0 0]  RotationSequenceAnglesUnits=deg  RotationMatrix=[1 0 0;0 1 0;0 0 1]  Quaternion=[1 0 0 0]  TranslationMethod=Cartesian  TranslationCartesianOffset=[params.f 0 0]  TranslationCartesianOffsetUnits=mm  TranslationStandardAxis=+Z  TranslationStandardOffset=0  TranslationStandardOffsetUnits=m  TranslationROffset=0  TranslationROffsetUnits=m  TranslationThetaOffset=0  TranslationThetaOffsetUnits=deg  TranslationZOffset=0  TranslationZOffsetUnits=m
  Rigid Transform9 : sm_lib/Frames and Transforms/Rigid Transform  RotationMethod=None  FollAlignAxisA=+X  BaseAlignAxisA=+Y  FollAlignAxisB=+Y  BaseAlignAxisB=+Z  RotationStandardAxis=+Z  RotationAngle=0  RotationAngleUnits=deg  RotationArbitraryAxis=[0 0 1]  RotationSequenceAxes=FollowerAxes  RotationSequence=XYX  RotationSequenceAngles=[0 0 0]  RotationSequenceAnglesUnits=deg  RotationMatrix=[1 0 0;0 1 0;0 0 1]  Quaternion=[1 0 0 0]  TranslationMethod=Cartesian  TranslationCartesianOffset=[params.f 0 0]  TranslationCartesianOffsetUnits=mm  TranslationStandardAxis=+Z  TranslationStandardOffset=0  TranslationStandardOffsetUnits=m  TranslationROffset=0  TranslationROffsetUnits=m  TranslationThetaOffset=0  TranslationThetaOffsetUnits=deg  TranslationZOffset=0  TranslationZOffsetUnits=m
  Solver Configuration : nesl_utility/Solver Configuration  PhysicalDomain=network_engine_domain  SubClassName=solver  LeftPortType=input  RightPortType=generic  Tones=[]  Harmonics=[]  SimulateNoise=off  Profile=off  UseLocalSampling=off  EnableSwitchedLinearOptims=on  FrequencyDomain=off  UseCCode=off  RelTol=0.001  AbsTol=0.001  MinStep=1e-09  ToWorkspace=off  RevertToSquareIcSolve=off  NumHomotopyIterations=100  PhasorMode=off  PhasorModeNumHarmonics=1  ConsistencySolver=NEWTON_XTOL_AFTER_FTOL  CanonicalOrdering=CANONICAL  OptimizeIntermediates=OPTIMIZED  IndexReductionMethod=DerivativeReplacement  DoDC=off  ResidualTolerance=1e-09  ConsistencyTolSource=GLOBAL  ConsistencyAbsTol=0.001  ConsistencyRelTol=0.001  ConsistencyTolFactor=0.001  UseLocalSolver=off  LocalSolverChoice=NE_BACKWARD_EULER_ADVANCER  ResolveIndetEquations=on  FunctionEvalNumThread=1  LocalSolverSampleTime=0.001  DoFixedCost=off  MaxNonlinIter=3  MaxModeIter=2  ComputeImpulses=off  ImpulseIterations=2  LinearAlgebra=auto  LinearAlgebraNumThread=0  EquationFormulation=NE_TIME_EF  DelaysMemoryBudget=1024  AutomaticFiltering=on  FilteringTimeConstant=0.001  PartitionStorageMethod=AS_NEEDED  PartitionMemoryBudget=1024  PartitionMethod=ROBUST  MultibodyUseLocalSolver=off  MultibodyLocalSolverChoice=ODE1  MultibodyLocalSolverSampleTime=0.001
  Subsystem1 : Subsystem  ReferencedSubsystem=R_Trident_Arm
  Subsystem2 : Subsystem  ReferencedSubsystem=R_Trident_Arm
  Subsystem3 : Subsystem  ReferencedSubsystem=R_Trident_Arm
  Transform Sensor : sm_lib/Frames and Transforms/Transform Sensor  MeasurementFrame=World  RotationSequence=XYX  SenseAngle=off  SenseAxis=off  SenseQ=off  SenseR=off  SenseRotationSequence=off  SenseOmegaX=off  SenseOmegaY=off  SenseOmegaZ=off  SenseOmega=off  SenseQDot=off  SenseRDot=off  SenseRotationSequenceDot=off  SenseAlphaX=off  SenseAlphaY=off  SenseAlphaZ=off  SenseAlpha=off  SenseQDDot=off  SenseRDDot=off  SenseX=on  SenseY=on  SenseZ=on  SenseXYZ=off  SenseRad=off  SenseAzim=off  SenseDist=off  SenseInc=off  SenseXDot=off  SenseYDot=off  SenseZDot=off  SenseXYZDot=off  SenseRadDot=off  SenseAzimDot=off  SenseDistDot=off  SenseIncDot=off  SenseXDDot=off  SenseYDDot=off  SenseZDDot=off  SenseXYZDDot=off  SenseRadDDot=off  SenseAzimDDot=off  SenseDistDDot=off  SenseIncDDot=off
  Transform Sensor1 : sm_lib/Frames and Transforms/Transform Sensor  MeasurementFrame=World  RotationSequence=XYX  SenseAngle=off  SenseAxis=off  SenseQ=off  SenseR=off  SenseRotationSequence=off  SenseOmegaX=off  SenseOmegaY=off  SenseOmegaZ=off  SenseOmega=off  SenseQDot=off  SenseRDot=off  SenseRotationSequenceDot=off  SenseAlphaX=off  SenseAlphaY=off  SenseAlphaZ=off  SenseAlpha=off  SenseQDDot=off  SenseRDDot=off  SenseX=on  SenseY=on  SenseZ=on  SenseXYZ=off  SenseRad=off  SenseAzim=off  SenseDist=off  SenseInc=off  SenseXDot=on  SenseYDot=on  SenseZDot=on  SenseXYZDot=off  SenseRadDot=off  SenseAzimDot=off  SenseDistDot=off  SenseIncDot=off  SenseXDDot=on  SenseYDDot=on  SenseZDDot=on  SenseXYZDDot=off  SenseRadDDot=off  SenseAzimDDot=off  SenseDistDDot=off  SenseIncDDot=off
  World Frame : sm_lib/Frames and Transforms/World Frame
  PositionMot1 : Outport
  Position2Mot2 : Outport  Port=2
  PositionMot3 : Outport  Port=3
  PositionXYZ : Outport  Port=4
  ForceJoint : Outport  Port=5
  Pos_EndEff : Outport  Port=6
  V_EndEff : Outport  Port=7
  A_EndEff : Outport  Port=8
  Arm1_qwb : Outport  Port=9
  Arm2_qwb : Outport  Port=10
  Arm3_qwb : Outport  Port=11
  wires:
  PS-Simulink Converter2/1 -> Mux1/3
  PS-Simulink Converter/1 -> Mux1/1
  Subsystem1/1 -> Position2Mot2/1
  PS-Simulink Converter1/1 -> Mux1/2
  Mux1/1 -> PositionXYZ/1
  Subsystem2/1 -> PositionMot3/1
  T_in1/1 -> Subsystem1/1
  T_in2/1 -> Subsystem2/1
  T_in/1 -> Subsystem3/1
  Subsystem3/1 -> PositionMot1/1
  Subsystem3/2 -> ForceJoint/1
  PS-Simulink Converter3/1 -> Gain/1
  PS-Simulink Converter4/1 -> Gain1/1
  PS-Simulink Converter5/1 -> Gain2/1
  PS-Simulink Converter6/1 -> Mux2/1
  PS-Simulink Converter7/1 -> Mux2/2
  PS-Simulink Converter8/1 -> Mux2/3
  PS-Simulink Converter9/1 -> Mux3/1
  PS-Simulink Converter10/1 -> Mux3/2
  PS-Simulink Converter11/1 -> Mux3/3
  Mux/1 -> Pos_EndEff/1
  Mux2/1 -> V_EndEff/1
  Mux3/1 -> A_EndEff/1
  Subsystem3/3 -> Arm1_qwb/1
  Subsystem1/2 -> Arm2_qwb/1
  Subsystem2/2 -> Arm3_qwb/1
  Gain/1 -> Mux/1
  Gain1/1 -> Mux/2
  Gain2/1 -> Mux/3
  connections:
  Rigid Transform2/LConn1 -- Subsystem1/RConn1
  Subsystem1/LConn1 -- Rigid Transform8/RConn1
  Transform Sensor/RConn3 -- PS-Simulink Converter1/LConn1
  Rigid Transform9/RConn1 -- Subsystem2/LConn1
  Rigid Transform6/LConn1 -- Rigid Transform12/RConn1
  Transform Sensor/LConn1 -- World Frame/RConn1 -- Rigid Transform10/LConn1 -- Solver Configuration/RConn1 -- Rigid Transform12/LConn1 -- Mechanism Configuration/RConn1 -- Rigid Transform11/LConn1 -- Transform Sensor1/LConn1
  PS-Simulink Converter2/LConn1 -- Transform Sensor/RConn4
  Rigid Transform5/LConn1 -- Subsystem2/RConn1
  Rigid Transform4/RConn1 -- Rigid Transform7/LConn1
  Rigid Transform9/LConn1 -- Rigid Transform6/RConn1
  Rigid Transform3/LConn1 -- Rigid Transform11/RConn1
  PS-Simulink Converter/LConn1 -- Transform Sensor/RConn2
  Rigid Transform3/RConn1 -- Rigid Transform8/LConn1
  Rigid Transform5/RConn1 -- End-effector/LConn1 -- Transform Sensor1/RConn1 -- Transform Sensor/RConn1 -- Rigid Transform1/RConn1 -- Rigid Transform2/RConn1
  Rigid Transform10/RConn1 -- Rigid Transform4/LConn1
  Subsystem3/LConn1 -- Rigid Transform7/RConn1
  Subsystem3/RConn1 -- Rigid Transform1/LConn1
  PS-Simulink Converter5/LConn1 -- Transform Sensor1/RConn4
  Transform Sensor1/RConn5 -- PS-Simulink Converter6/LConn1
  PS-Simulink Converter7/LConn1 -- Transform Sensor1/RConn6
  Transform Sensor1/RConn7 -- PS-Simulink Converter8/LConn1
  Transform Sensor1/RConn8 -- PS-Simulink Converter9/LConn1
  Transform Sensor1/RConn9 -- PS-Simulink Converter10/LConn1
  Transform Sensor1/RConn10 -- PS-Simulink Converter11/LConn1
  Transform Sensor1/RConn3 -- PS-Simulink Converter3/LConn1
  Transform Sensor1/RConn2 -- PS-Simulink Converter4/LConn1

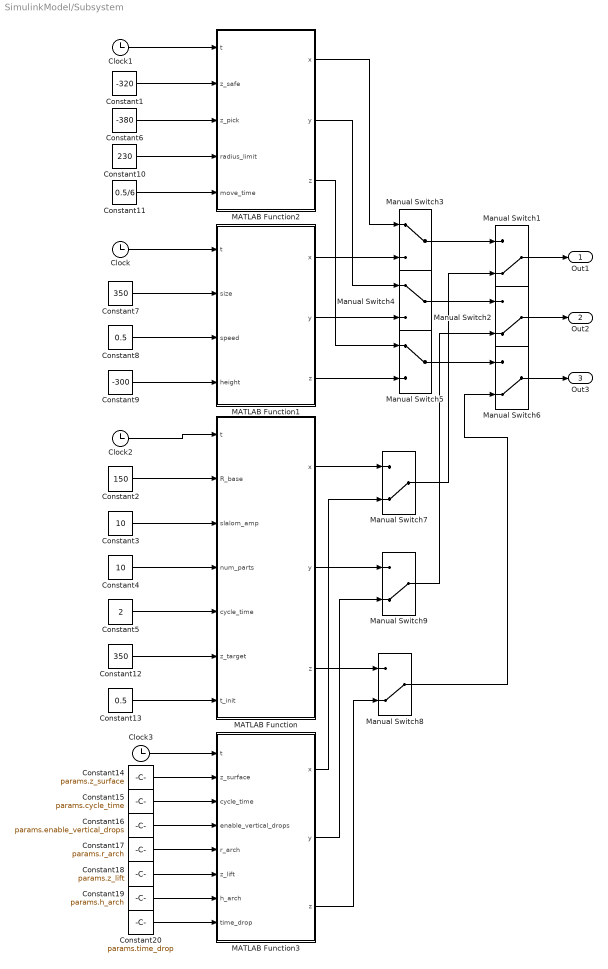
== system SimulinkModel/Subsystem ==
  Clock{,1..3} (4 alike) : Clock
  Constant1 : Constant  Value=-320
  Constant10 : Constant  Value=230
  Constant11 : Constant  Value=0.5/6
  Constant12 : Constant  Value=350
  Constant13 : Constant  Value=0.5
  Constant14 : Constant  Value=params.z_surface
  Constant15 : Constant  Value=params.cycle_time
  Constant16 : Constant  Value=params.enable_vertical_drops
  Constant17 : Constant  Value=params.r_arch
  Constant18 : Constant  Value=params.z_lift
  Constant19 : Constant  Value=params.h_arch
  Constant2 : Constant  Value=150
  Constant20 : Constant  Value=params.time_drop
  Constant3 : Constant  Value=10
  Constant4 : Constant  Value=10
  Constant5 : Constant  Value=2
  Constant6 : Constant  Value=-380
  Constant7 : Constant  Value=350
  Constant8 : Constant  Value=0.5
  Constant9 : Constant  Value=-300
  MATLAB Function : MATLAB Function  TreatAsAtomicUnit=on
  MATLAB Function1 : MATLAB Function  TreatAsAtomicUnit=on
  MATLAB Function2 : MATLAB Function  TreatAsAtomicUnit=on
  MATLAB Function3 : MATLAB Function  TreatAsAtomicUnit=on
  Manual Switch{1..2,6..9} (6 alike) : ManualSwitch  CurrentSetting=0
  Manual Switch3 : ManualSwitch
  Manual Switch4 : ManualSwitch
  Manual Switch5 : ManualSwitch
  Out1 : Outport
  Out2 : Outport  Port=2
  Out3 : Outport  Port=3
  wires:
  Constant9/1 -> MATLAB Function1/4(height)
  Constant11/1 -> MATLAB Function2/5(move_time)
  Constant6/1 -> MATLAB Function2/3(z_pick)
  Constant1/1 -> MATLAB Function2/2(z_safe)
  MATLAB Function2/2(y) -> Manual Switch4/1
  MATLAB Function2/3(z) -> Manual Switch5/1
  Constant8/1 -> MATLAB Function1/3(speed)
  Clock/1 -> MATLAB Function1/1(t)
  Constant7/1 -> MATLAB Function1/2(size)
  Constant10/1 -> MATLAB Function2/4(radius_limit)
  Clock1/1 -> MATLAB Function2/1(t)
  MATLAB Function1/1(x) -> Manual Switch3/2
  MATLAB Function2/1(x) -> Manual Switch3/1
  MATLAB Function1/2(y) -> Manual Switch4/2
  MATLAB Function1/3(z) -> Manual Switch5/2
  Clock2/1 -> MATLAB Function/1(t)
  Constant2/1 -> MATLAB Function/2(R_base)
  Constant4/1 -> MATLAB Function/4(num_parts)
  Constant3/1 -> MATLAB Function/3(slalom_amp)
  Constant5/1 -> MATLAB Function/5(cycle_time)
  Constant12/1 -> MATLAB Function/6(z_target)
  Constant13/1 -> MATLAB Function/7(t_init)
  Manual Switch3/1 -> Manual Switch1/1
  Manual Switch4/1 -> Manual Switch2/1
  Manual Switch5/1 -> Manual Switch6/1
  Manual Switch6/1 -> Out3/1
  Manual Switch2/1 -> Out2/1
  Manual Switch1/1 -> Out1/1
  Clock3/1 -> MATLAB Function3/1(t)
  Constant14/1 -> MATLAB Function3/2(z_surface)
  Constant15/1 -> MATLAB Function3/3(cycle_time)
  MATLAB Function/1(x) -> Manual Switch7/1
  MATLAB Function/2(y) -> Manual Switch9/1
  MATLAB Function/3(z) -> Manual Switch8/1
  MATLAB Function3/1(x) -> Manual Switch7/2
  Manual Switch7/1 -> Manual Switch1/2
  Manual Switch9/1 -> Manual Switch2/2
  Manual Switch8/1 -> Manual Switch6/2
  MATLAB Function3/2(y) -> Manual Switch9/2
  MATLAB Function3/3(z) -> Manual Switch8/2
  Constant16/1 -> MATLAB Function3/4(enable_vertical_drops)
  Constant19/1 -> MATLAB Function3/7(h_arch)
  Constant18/1 -> MATLAB Function3/6(z_lift)
  Constant17/1 -> MATLAB Function3/5(r_arch)
  Constant20/1 -> MATLAB Function3/8(time_drop)

== matlab function SimulinkModel/Subsystem/MATLAB Function1 ==
  data: x output; t input; y output; size input; speed input; height input; z output
function [x, y, z] = square_path(t, size, speed, height)
    % t: simulation time
    % size: 300
    % speed: 0.5 (Hz) - how fast it completes a lap
    % height: -400
    
    half = size / 2;
    period = 1/speed;
    pos = mod(t, period) / period; % 0 to 1 progress of the lap
    
    if pos < 0.25
        % Top edge
        x = half - (pos/0.25)*size;
        y = half;
    elseif pos < 0.50
        % Left edge
        x = -half;
        y = half - ((pos-0.25)/0.25)*size;
    elseif pos < 0.75
        % Bottom edge
        x = -half + ((pos-0.50)/0.25)*size;
        y = -half;
    else
        % Right edge
        x = half;
        y = -half + ((pos-0.75)/0.25)*size;
    end
    
    z = height;
end

== matlab function SimulinkModel/MATLAB Function ==
  data: x input; q1 output; y input; z input; f input; e input; L input; l input; q2 output; q3 output
function [q1, q2, q3] = fcn(x, y, z, f, e, L, l)

    % Calculate Radian outputs (0 = Vertical Down, 1.57 = Horizontal)
    q1 = solve_delta_rad(x, y, z, 0, f, e, L, l);
    q2 = solve_delta_rad(x, y, z, 120, f, e, L, l);
    q3 = solve_delta_rad(x, y, z, 240, f, e, L, l);
end

function q = solve_delta_rad(px, py, pz, phi_deg, f, e, L, l)
    % 1. Rotate Cartesian coordinates into the arm's local coordinate frame
    phi = phi_deg * (pi/180);
    X = px * cos(phi) + py * sin(phi);
    Y = -px * sin(phi) + py * cos(phi) + (f - e);
    Z = pz;

    % 2. Set up the exact 3D sphere-intersection equation
    % This represents A*cos(q) + B*sin(q) = C
    A = 2 * L * Z;
    B = 2 * L * Y;
    C = l^2 - L^2 - X^2 - Y^2 - Z^2;

    % 3. Check for physical reachability (prevent imaginary numbers)
    discriminant = A^2 + B^2 - C^2;
    if discriminant < 0
        % Target is physically unreachable, return a safe hold position
        q = 0.1; 
        return;
    end

    % 4. Solve the quadratic equation using tangent half-angle substitution
    % The minus root gives the standard "elbow pointing outwards" configuration
    t = (B - sqrt(discriminant)) / (A + C);
    
    % Calculate final angle
    q = 2 * atan(t);

    % 5. Enforce mechanical limits (Degrees to Radians)
    if q > 2.0
        q = 2.0; 
    elseif q < 0.1
        q = 0.1; 
    end 
end

== matlab function SimulinkModel/Subsystem/MATLAB Function2 ==
  settings: updateMethod=DISCRETE  sampleTime=0.001
  data: x output; t input; y output; z_safe input; z_pick input; radius_limit input; z output; move_time input
function [x, y, z] = fcn(t, z_safe, z_pick, radius_limit, move_time)
    % t: Simulation clock
    % z_safe: Travel height (e.g., -350)
    % z_pick: Surface height (e.g., -500)
    % radius_limit: Max XY distance from center (e.g., 100)
    % move_time: Seconds per move (e.g., 2.0)

    persistent target_pos start_pos move_start_time phase
    
    % Initialize
    if isempty(target_pos)
        target_pos = [0, 0, z_safe];
        start_pos = [0, 0, z_safe];
        move_start_time = 0;
        phase = 0; % 0: Move Up, 1: Move XY, 2: Move Down
    end

    % Check if it's time for a new random target
    elapsed = t - move_start_time;
    
    if elapsed >= move_time
        move_start_time = t;
        start_pos = target_pos;
        
        % Generate a new random XY within a circle
        angle = rand() * 2 * pi;
        r = rand() * radius_limit;
        new_x = r * cos(angle);
        new_y = r * sin(angle);
        
        % Toggle between picking down and moving safe
        if phase == 0 % Just moved up, now move XY
            target_pos = [new_x, new_y, z_safe];
            phase = 1;
        elseif phase == 1 % Just moved XY, now move Down
            target_pos = [start_pos(1), start_pos(2), z_pick];
            phase = 2;
        else % Just moved Down, now move back Up
            target_pos = [start_pos(1), start_pos(2), z_safe];
            phase = 0;
        end
    end

    % Smooth Interpolation (S-Curve/Sine)
    % This prevents the "slams" by making velocity zero at start and end
    s = (1 - cos(pi * (t - move_start_time) / move_time)) / 2;
    
    x = start_pos(1) + s * (target_pos(1) - start_pos(1));
    y = start_pos(2) + s * (target_pos(2) - start_pos(2));
    z = start_pos(3) + s * (target_pos(3) - start_pos(3));
end

== matlab function SimulinkModel/MATLAB Function1 ==
  data: x output; q1 input; y output; q2 input; q3 input; f input; e input; L input; l input; z output
function [x, y, z] = fcn(q1, q2, q3, f, e, L, l)

phi1 = 0;
phi2 = 120 * (pi/180);
phi3 = 240 * (pi/180);


% Calculate effective radius of each elbow from the center
r1 = f - e - L * sin(q1);
r2 = f - e - L * sin(q2);
r3 = f - e - L * sin(q3);

% Elbow Cartesian coordinates
Ex1 = r1 * sin(phi1);
Ey1 = -r1 * cos(phi1);
Ez1 = -L * cos(q1);

Ex2 = r2 * sin(phi2);
Ey2 = -r2 * cos(phi2);
Ez2 = -L * cos(q2);

Ex3 = r3 * sin(phi3);
Ey3 = -r3 * cos(phi3);
Ez3 = -L * cos(q3);

% The end effector position is the intersection of 3 spheres 
% with radius l centered at the elbows.
% Differentiating the sphere equations yields two planes to find X and Y as a function of Z.

E1_sq = Ex1^2 + Ey1^2 + Ez1^2;
E2_sq = Ex2^2 + Ey2^2 + Ez2^2;
E3_sq = Ex3^2 + Ey3^2 + Ez3^2;

A1 = 2 * (Ex1 - Ex2);
B1 = 2 * (Ey1 - Ey2);
C1 = 2 * (Ez1 - Ez2);
D1 = E1_sq - E2_sq;

A2 = 2 * (Ex1 - Ex3);
B2 = 2 * (Ey1 - Ey3);
C2 = 2 * (Ez1 - Ez3);
D2 = E1_sq - E3_sq;

% Cramer's rule to find X and Y
den = A1 * B2 - A2 * B1;

if abs(den) < 1e-6
    % Safety constraint: Avoid division by zero if geometry collapses
    x = 0; y = 0; z = 0; 
    return;
end

ax = (D1 * B2 - D2 * B1) / den;
bx = (C2 * B1 - C1 * B2) / den;

ay = (A1 * D2 - A2 * D1) / den;
by = (A2 * C1 - A1 * C2) / den;

% Substitute back into Sphere 1 equation to solve for Z
x0 = ax - Ex1;
y0 = ay - Ey1;

a = bx^2 + by^2 + 1;
b = 2 * (x0 * bx + y0 * by - Ez1);
c = x0^2 + y0^2 + Ez1^2 - l^2;

delta = b^2 - 4 * a * c;

if delta < 0
    % Safety constraint: Angles provided are physically impossible (rods would disconnect)
    x = 0; y = 0; z = 0;
    return;
end

% Choose the negative root because the end effector is mounted below the motors
z = (-b - sqrt(delta)) / (2 * a);

% Calculate final X and Y
x = ax + bx * z;
y = ay + by * z;

== matlab function SimulinkModel/Subsystem/MATLAB Function ==
  data: x output; t input; y output; R_base input; slalom_amp input; num_parts input; cycle_time input; z_target input; t_init input; z output
function [x, y, z] = fcn(t, R_base, slalom_amp, num_parts, cycle_time, z_target, t_init)
    % t: Simulation clock (seconds)
    % R_base: Radius of the main circle (e.g., 100)
    % slalom_amp: Slalom weave depth (e.g., 20)
    % num_parts: Number of obstacles (e.g., 8)
    % cycle_time: Seconds per full lap (e.g., 5.0)
    % z_target: Constant Z depth (e.g., -350)
    % t_init: Time in seconds to slowly ramp up the motion (e.g., 2.0)

    % 1. Calculate the ideal moving path (The Slalom)
    theta = (t / cycle_time) * 2 * pi;
    R_dynamic = R_base + slalom_amp * sin(num_parts * theta);
    x_path = R_dynamic * cos(theta);
    y_path = R_dynamic * sin(theta);

    % 2. Generate the S-Curve Multiplier (0 to 1)
    if t <= t_init
        % Smooth half-cosine curve from 0 to 1
        s = (1 - cos(pi * t / t_init)) / 2;
    else
        % After initialization time expires, lock to 1 (full following)
        s = 1.0;
    end

    % 3. Apply the S-Curve to spiral outward from center
    % Assuming the robot's physical starting position is X=0, Y=0
    x_home = 0;
    y_home = 0;

    x = x_home + s * (x_path - x_home);
    y = y_home + s * (y_path - y_home);
    
    % Z stays flat the entire time
    z = z_target; 
end

== matlab function SimulinkModel/Subsystem/MATLAB Function3 ==
  settings: updateMethod=DISCRETE  sampleTime=0.001
  data: x output; t input; y output; z_surface input; cycle_time input; z output; enable_vertical_drops input; r_arch input; z_lift input; h_arch input; time_drop input
function [x, y, z] = fcn(t, z_surface, cycle_time, enable_vertical_drops, r_arch, z_lift, h_arch, time_drop)
    % Reachable parameters (now passed directly as inputs)
    R = r_arch;          
    t_init = 1.0;    % 1.0 second soft-start ramp from center
    
    phi0 = 0;
    xA0 = R * cos(phi0);
    yA0 = R * sin(phi0);
    
    % Phase 0: Jerk-limited soft startup from resting center
    if t < t_init
        u = t / t_init;
        s = u^3 * (10 - 15*u + 6*u^2); % 5th-Order Minimum Jerk Profile
        
        x = s * xA0;
        y = s * yA0;
        z = z_surface;
        return;
    end
    
    % Continuous sequence through the 6 diagonal chords
    t_run = t - t_init;
    
    % DYNAMIC CYCLE TIME LOGIC (-0.2s per full pattern)
    T_current = cycle_time; 
    t_accum = 0;            
    time_drop = time_drop;     
    
    for p = 1:100 
        T_pattern = 6 * T_current;
        if t_run < (t_accum + T_pattern)
            break;
        end
        t_accum = t_accum + T_pattern;
        T_current = max(0.05, T_current - time_drop); % Safeguard against negative or zero time
    end
    
    t_local = t_run - t_accum;
    cycle_idx = floor(t_local / T_current);
    diag_idx = mod(cycle_idx, 6);
    
    % Pick (A) and Place (B) angles (60 degree steps)
    phi_pick = diag_idx * (pi / 3);
    phi_place = phi_pick + pi;
    phi_next = (diag_idx + 1) * (pi / 3);
    
    xA = R * cos(phi_pick);
    yA = R * sin(phi_pick);
    xB = R * cos(phi_place);
    yB = R * sin(phi_place);
    xNext = R * cos(phi_next);
    yNext = R * sin(phi_next);
    
    % Progress within the current specific pick & place chord [0, 1]
    tau = mod(t_local, T_current) / T_current;
    
    if enable_vertical_drops == 1
        % ORIGINAL 4-PHASE: Stop and plunge vertically at endpoints
        if tau < 0.15
            u = tau / 0.15;
            s = u^3 * (10 - 15*u + 6*u^2);
            x = xA; y = yA; z = z_surface + s * z_lift;
        elseif tau < 0.65
            u = (tau - 0.15) / 0.50;
            s_xy = u^3 * (10 - 15*u + 6*u^2);
            x = xA + s_xy * (xB - xA); y = yA + s_xy * (yB - yA);
            z = z_surface + z_lift + h_arch * (sin(pi * u))^2;
        elseif tau < 0.80
            u = (tau - 0.65) / 0.15;
            s = u^3 * (10 - 15*u + 6*u^2);
            x = xB; y = yB; z = (z_surface + z_lift) - s * z_lift;
        else
            u = (tau - 0.80) / 0.20;
            s_tr = u^3 * (10 - 15*u + 6*u^2);
            x = xB + s_tr * (xNext - xB); y = yB + s_tr * (yNext - yB);
            z = z_surface + (z_lift + 10) * (sin(pi * u))^2;
        end
    else
        % CONTINUOUS MODE: Pure parabolic sweeping arches without vertical stops
        total_clearance = z_lift + h_arch;
        
        if tau < 0.50
            u = tau / 0.50;
            s_xy = u^3 * (10 - 15*u + 6*u^2);
            x = xA + s_xy * (xB - xA);
            y = yA + s_xy * (yB - yA);
            z = z_surface + total_clearance * (sin(pi * u))^2;
        else
            u = (tau - 0.50) / 0.50;
            s_tr = u^3 * (10 - 15*u + 6*u^2);
            x = xB + s_tr * (xNext - xB);
            y = yB + s_tr * (yNext - yB);
            z = z_surface + total_clearance * (sin(pi * u))^2;
        end
    end
end
